simulink model "mass2"  (R2022a)
settings: Solver=FixedStepAuto  StartTime=0.0  StopTime=20  FixedStep=2e-5  RelTol=1e-3
values from neighbouring files (symbols this model uses):
  J2 = 0.12    [EDriveLab1.m]
undefined symbols (not defined in the file or in its folder): J1, K12
settings Model: Creator=Family  LastModifiedBy=Family

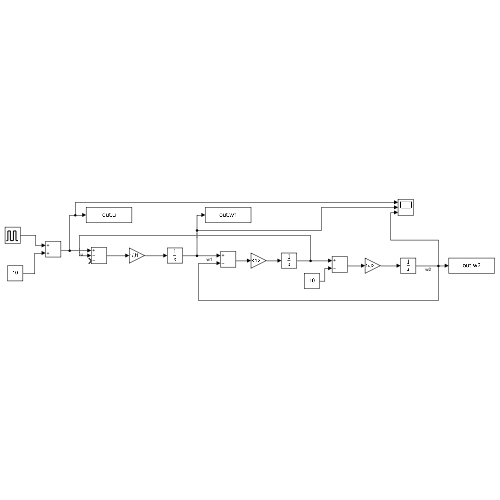
[thumbnail: Simulink's stored preview of the top-level diagram]
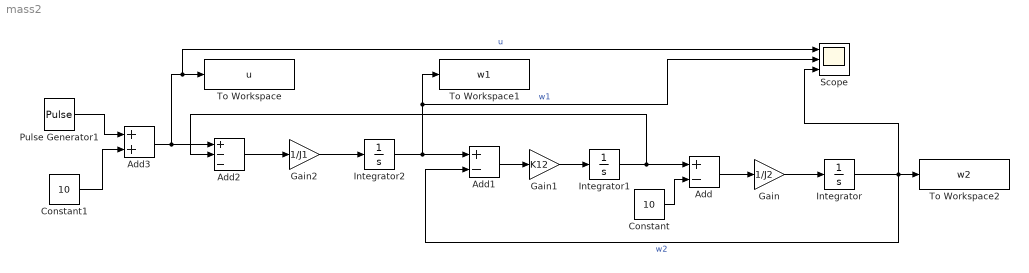
== system mass2 ==
  Add : Sum  Inputs=+-
  Add1 : Sum  Inputs=+-
  Add2 : Sum  Inputs=+--
  Add3 : Sum
  Constant : Constant  Value=10
  Constant1 : Constant  Value=10
  Gain : Gain  Gain=1/J2
  Gain1 : Gain  Gain=K12
  Gain2 : Gain  Gain=1/J1
  Integrator : Integrator
  Integrator1 : Integrator
  Integrator2 : Integrator
  Pulse Generator1 : DiscretePulseGenerator  PulseType=Time based  Amplitude=10  Period=5  PulseWidth=50
  Scope : Scope  NumInputPorts=3
  To Workspace : ToWorkspace  VariableName=u  SaveFormat=Timeseries  SampleTime=0.001
  To Workspace1 : ToWorkspace  VariableName=w1  SaveFormat=Timeseries  SampleTime=0.001
  To Workspace2 : ToWorkspace  VariableName=w2  SaveFormat=Timeseries  SampleTime=0.001
  wires:
  Gain/1 -> Integrator/1
  Add/1 -> Gain/1
  Integrator1/1 -> Add/1, Add2/2
  Gain1/1 -> Integrator1/1
  Add1/1 -> Gain1/1
  Integrator/1 -> Scope/3, Add1/2, To Workspace2/1  "w2"
  Integrator2/1 -> Add1/1, Scope/2, To Workspace1/1  "w1"
  Gain2/1 -> Integrator2/1
  Add2/1 -> Gain2/1
  Constant/1 -> Add/2
  Add3/1 -> Add2/1, Scope/1, To Workspace/1  "u"
  Pulse Generator1/1 -> Add3/1
  Constant1/1 -> Add3/2
